simulink model "STEP1_W"  (Simulink 8.4)
settings: Solver=ode45  SolverMode=SingleTasking  StartTime=0.0  StopTime=inf  FixedStep=2/64e5  RelTol=1e-3
values from neighbouring files (symbols this model uses):
  c = (U_E025^2-U_ES^2)/U_NG025^2    [Digital_AM_SNR_to_BER.m]    (also in KOSZI_P.m = menu('Kanalwahl','1-Kanal','2-Kanal','3-Kanal'); exercise_00.m = 300000000)
libraries: measurement_tools x5, system_blocks x2, dsparch4 x2, dspvision x2, dspmtrx3 x1, dspsnks4 x1
settings Model: Creator=Schoenen  LastModifiedBy=Schoenen
settings DataIOCC: SignalLoggingName=sigsOut
settings OptimizationCC: ExpressionDepthLimit=128
settings DebuggingCC: SaveWithParameterizedLinksMsg=none  SignalResolutionControl=TryResolveAllWithWarning  SolverPrmCheckMsg=none  MultiTaskDSMMsg=warning  MultiTaskCondExecSysMsg=none  FcnCallInpInsideContextMsg=EnableAllAsError  StateNameClashWarn=none
settings HardwareCC: TargetLongLongMode=on  TargetIntDivRoundTo=Zero  TargetEndianess=LittleEndian  TargetHWDeviceType=MATLAB Host  ProdEqTarget=off
settings RTWCC: IncludeERTFirstTime=on

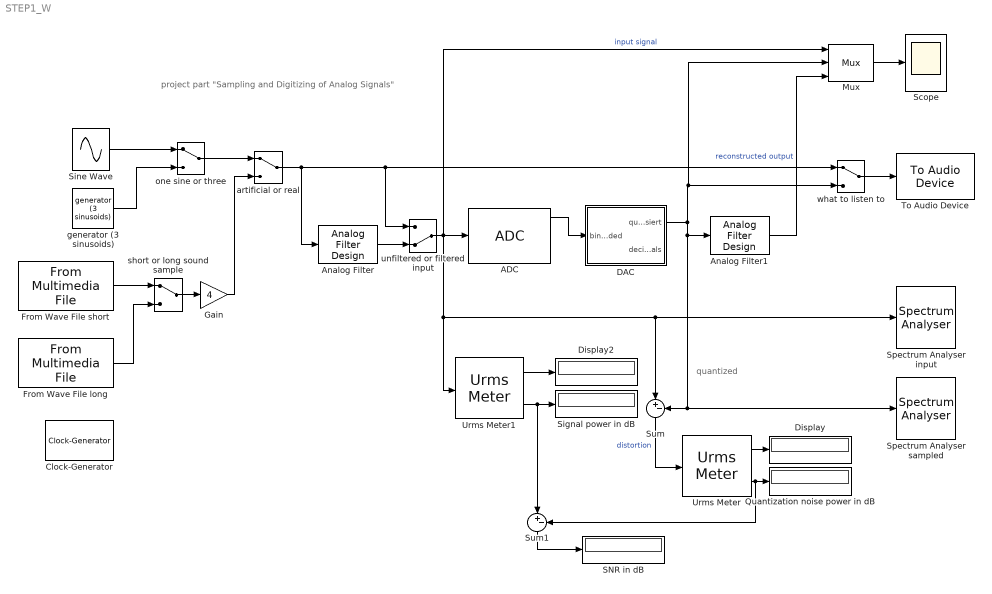
== system STEP1_W ==
  note: quantized
  note: project part "Sampling and Digitizing of Analog Signals"
  ADC : system_blocks/ADC  umax=1  bits=c.bit_resolution  bipolar=off
  Analog Filter : dsparch4/Analog Filter Design  method=Butterworth  filttype=Lowpass  N=24  Wlo=2*pi*c.filter_cutoff_frequency  Whi=80  Rp=2  Rs=40
  Analog Filter1 : dsparch4/Analog Filter Design  method=Butterworth  filttype=Lowpass  N=24  Wlo=2*pi*c.filter_cutoff_frequency  Whi=80  Rp=2  Rs=40
  Clock-Generator : system_blocks/Clock-Generator  bt=c.bit_clock_frequency  sr=c.sampling_frequency
  DAC : Subsystem  AncestorBlock=system_blocks/DAC  mask(Digital-Analog-Converter (DAC)){umax=1, bits=c.bit_resolution, bipolar=off}
      mask prompts: umax "maximum voltage limit:"; bits "number of bits (1...16):"; bipolar "bipolare binary input sequence:"
      mask help:
      | Der DAC wandelt ein binäres Digitalsignal (PCM) in ein bipolares, quantisiertes Analogsignal mit den Austeuergrenzen +/- Umax um.
      |
      | Eingang :              Bit-Paralleleingang, Binäre PCM-Zahlenfolge, je Abtastwert ein Zeilenvektor in Binärdarstellung
      |
      | Oberer  Ausgang:   Quantisiertes, bipolares Signal, begrenzt auf +/- Umax,  je Abtastwert ein als Skalar
      |
      | Unterer Ausgang:   dem Eingang entsprechender positiver  Dezimalwert im Bereich 0.... 2^bits -1
      mask Help:
      | Author: Prof. Dr.-Ing. Peter Kröger
      | copyright 2002
      | <p>
      | 
      | Der DAC wandelt ein binäres Digitalsignal (PCM) in ein bipolares, quantisiertes Analogsignal mit den Austeuergrenzen +/- Umax um.
      | <p>
      | Eingang :                Binäre PCM-Zahlenfolge, je Abtastwert ein Zeilenvektor in
      |                                Binärdarstellung
      | <p>
      | Oberer  Ausgang:   Quantisiertes, bipolares Signal, begrenzt auf +/- Umax,
      |                                je Abtastwert ein als Skalar
      | <p>
      | Unterer Ausgang:   dem Eingang entsprechender positiver  Dezimalwert
      |                                im Bereich 0.... 2^bits -1
  Display : Display
      settings: Format=short_e
  Display2 : Display
      settings: Format=short_e
  From Wave File long : dspvision/From Multimedia File  inputFilename=audio_sampled_with_8kHz.wav  loop=on  numPlays=1  outputStreams=Audio only  videoDataType=single  audioDataType=double  inheritSampleTime=on  userDefinedSampleTime=1/30  noAudioOutput=off  isIntensityVideo=off  fourcc=RGB  colorVideoFormat=Separate color signals  outputEOF=off  dataOrg=Column-major  audioFrameSize=1  computeAudioFrameSize=off  outSamplingMode=Sample based
  From Wave File short : dspvision/From Multimedia File  inputFilename=audio_in_8kHz.wav  loop=on  numPlays=1  outputStreams=Audio only  videoDataType=single  audioDataType=double  inheritSampleTime=on  userDefinedSampleTime=1/30  noAudioOutput=off  isIntensityVideo=off  fourcc=RGB  colorVideoFormat=Separate color signals  outputEOF=off  dataOrg=Column-major  audioFrameSize=1  computeAudioFrameSize=off  outSamplingMode=Sample based
  Gain : Gain  Gain=4
  Mux : Mux  Inputs=3
  Quantization noise power in dB : Display
      settings: Decimation=2
  SNR in dB : Display
      settings: Decimation=2
  Scope : Scope
      settings: TimeRange=1  YMin=-1.5  YMax=2
  Signal power in dB : Display
      settings: Decimation=2
  Sine Wave : Sin  Frequency=2*pi*1000  SampleTime=0
  Spectrum Analyser input : measurement_tools/Spectrum Analyser  st=c.sample_time
  Spectrum Analyser sampled : measurement_tools/Spectrum Analyser  st=c.sample_time/4
  Sum : Sum  Inputs=|+-
  Sum1 : Sum  Inputs=|+-
  To Audio Device : dspsnks4/To Audio Device  deviceName=Default  inheritSampleRate=off  sampleRate=8000  deviceDatatype=Determine from input data type  autoBufferSize=on  bufferSize=4096  queueDuration=1.0  defaultOutputChannelMapping=on  outputChannelMapping=1:2  outputNumUnderrunSamples=off
  Urms Meter : measurement_tools/Urms Meter  T=1
  Urms Meter1 : measurement_tools/Urms Meter  T=1
  artificial or real : ManualSwitch
  generator (3 sinusoids) : measurement_tools/generator (3 sinusoids)  MaskParam1="[1  1000  0]"  MaskParam2="[0.5  2000  0]"  MaskParam3="[0.25  3000  0]"
  one sine or three : ManualSwitch
  short or long sound sample : ManualSwitch
  unfiltered or filtered input : ManualSwitch  CurrentSetting=0
  what to listen to : ManualSwitch
  wires:
  Sine Wave/1 -> one sine or three/1
  generator (3 sinusoids)/1 -> one sine or three/2
  one sine or three/1 -> artificial or real/1
  From Wave File short/1 -> short or long sound sample/1
  From Wave File long/1 -> short or long sound sample/2
  artificial or real/1 -> what to listen to/1, unfiltered or filtered input/1, Analog Filter/1
  what to listen to/1 -> To Audio Device/1
  Analog Filter/1 -> unfiltered or filtered input/2
  unfiltered or filtered input/1 -> ADC/1, Sum/1, Spectrum Analyser input/1, Urms Meter1/1, Mux/1  "input signal"
  Mux/1 -> Scope/1
  Analog Filter1/1 -> Mux/3  "reconstructed output"
  short or long sound sample/1 -> Gain/1
  Gain/1 -> artificial or real/2
  ADC/1 -> DAC/1(binary_coded)
  DAC/1(quantisiert) -> Mux/2, what to listen to/2, Sum/2, Spectrum Analyser sampled/1, Analog Filter1/1
  Sum/1 -> Urms Meter/1  "distortion"
  Urms Meter/1 -> Display/1
  Urms Meter/2 -> Sum1/2, Quantization noise power in dB/1
  Urms Meter1/1 -> Display2/1
  Urms Meter1/2 -> Sum1/1, Signal power in dB/1
  Sum1/1 -> SNR in dB/1

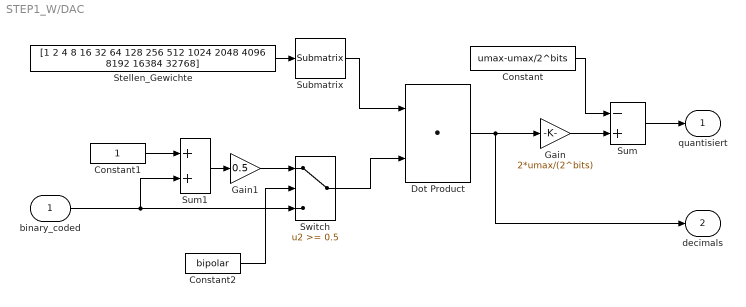
== system STEP1_W/DAC ==
  binary_coded : Inport
  Constant : Constant  Value=umax-umax/2^bits
  Constant1 : Constant
  Constant2 : Constant  Value=bipolar
  Dot Product : DotProduct  InputSameDT=on  OutDataTypeStr=Inherit: Inherit via internal rule
  Gain : Gain  Gain=2*umax/(2^bits)  SaturateOnIntegerOverflow=on  OutDataTypeStr=Inherit: Same as input  ParamDataTypeStr=Inherit: Same as input
  Gain1 : Gain  Gain=0.5  SaturateOnIntegerOverflow=on  OutDataTypeStr=Inherit: Same as input  ParamDataTypeStr=Inherit: Same as input
  Stellen_Gewichte : Constant  Value=[1 2 4 8 16 32 64 128 256 512 1024 2048 4096 8192 16384 32768]
  Submatrix : dspmtrx3/Submatrix  RowSpan=Range of rows  RowStartMode=First  RowStartIndex=1  RowEndMode=Index  RowEndIndex=bits  ColSpan=Range of columns  ColStartMode=First  ColStartIndex=1  ColEndMode=Last  ColEndIndex=bits-1
  Sum : Sum  Inputs=-+  SaturateOnIntegerOverflow=on  InputSameDT=on  OutDataTypeStr=Inherit: Same as first input
  Sum1 : Sum  SaturateOnIntegerOverflow=on  InputSameDT=on  OutDataTypeStr=Inherit: Same as first input
  Switch : Switch  Threshold=0.5  SaturateOnIntegerOverflow=on  InputSameDT=on
  quantisiert : Outport
  decimals : Outport  Port=2
  wires:
  Stellen_Gewichte/1 -> Submatrix/1
  Submatrix/1 -> Dot Product/1
  Constant/1 -> Sum/1
  Sum/1 -> quantisiert/1
  Dot Product/1 -> decimals/1, Gain/1
  Gain/1 -> Sum/2
  Switch/1 -> Dot Product/2
  binary_coded/1 -> Switch/3, Sum1/2
  Constant1/1 -> Sum1/1
  Sum1/1 -> Gain1/1
  Gain1/1 -> Switch/1
  Constant2/1 -> Switch/2
